simulink model "dynamics_bicycle_model"  (R2017b)
settings: Solver=FixedStepAuto  StartTime=0.0  StopTime=5  FixedStep=0.002  RelTol=1e-3
values from neighbouring files (symbols this model uses):
  af = 1.07    [main_dynamic_bicycle.m]
  ar = 0.936    [main_dynamic_bicycle.m]
  Bf = 0.242    [main_dynamic_bicycle.m]
  Br = 0.24    [main_dynamic_bicycle.m]
  Cf = 1.352    [main_dynamic_bicycle.m]
  Cr = 1.29    [main_dynamic_bicycle.m]
  Df = 2751.69    [main_dynamic_bicycle.m]
  Dr = 3113.08    [main_dynamic_bicycle.m]
  Ef = -0.392    [main_dynamic_bicycle.m]
  Er = 0.507    [main_dynamic_bicycle.m]
  input_type = 3    [main_bicycle.m]    (also in main_differential_steer.m; main_dynamic_bicycle.m)
  Iz = 552.718    [main_dynamic_bicycle.m]
  m = 645    [main_dynamic_bicycle.m]
  r = 0.3    [main_dynamic_bicycle.m]
  theta0 = 0    [main_differential_steer.m]    (also in main_dynamic_bicycle.m)
  v_const = 1    [main_bicycle.m]    (also in main_dynamic_bicycle.m = 0.9)
  v_dot = 0    [main_dynamic_bicycle.m]
  x0 = 0    [main_differential_steer.m]    (also in main_dynamic_bicycle.m)
  y0 = 0    [main_differential_steer.m]    (also in main_dynamic_bicycle.m)
settings Model: Creator=zhenghe3  LastModifiedBy=zhenghe3

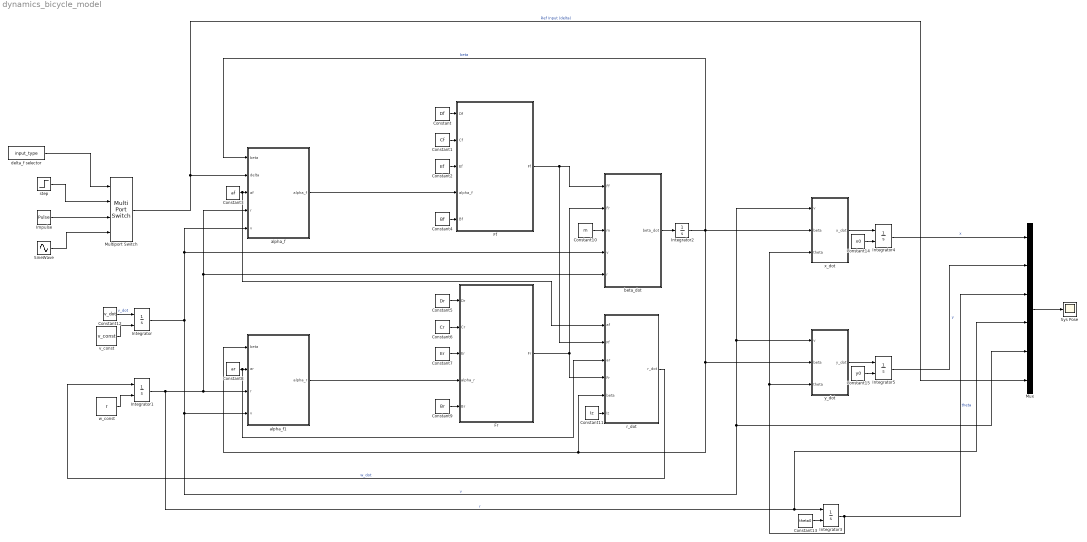
== system dynamics_bicycle_model ==
  Constant : Constant  Value=Df
  Constant1 : Constant  Value=Cf
  Constant10 : Constant  Value=m
  Constant11 : Constant  Value=Iz
  Constant12 : Constant  Value=v_dot
  Constant13 : Constant  Value=theta0
  Constant14 : Constant  Value=x0
  Constant15 : Constant  Value=y0
  Constant2 : Constant  Value=Ef
  Constant3 : Constant  Value=af
  Constant4 : Constant  Value=Bf
  Constant5 : Constant  Value=Dr
  Constant6 : Constant  Value=Cr
  Constant7 : Constant  Value=Er
  Constant8 : Constant  Value=ar
  Constant9 : Constant  Value=Br
  Ff : MATLAB Function  TreatAsAtomicUnit=on
  Fr : MATLAB Function  TreatAsAtomicUnit=on
  Impulse : DiscretePulseGenerator  PulseType=Time based  Period=1  PulseWidth=50
  Integrator{,1,3..5} (5 alike) : Integrator  InitialConditionSource=external
  Integrator2 : Integrator
  Multiport Switch : MultiPortSwitch
  Mux : Mux  Inputs=6
  SineWave : Sin  Frequency=5  SampleTime=0
  Sys Pose : Scope
  alpha_f : MATLAB Function  TreatAsAtomicUnit=on
  alpha_f1 : MATLAB Function  TreatAsAtomicUnit=on
  beta_dot : MATLAB Function  TreatAsAtomicUnit=on
  delta_f selector : Constant  Value=input_type
  r_dot : MATLAB Function  TreatAsAtomicUnit=on
  step : Step  Time=0  SampleTime=0
  v_const : Constant  Value=v_const
  w_const : Constant  Value=r
  x_dot : MATLAB Function  TreatAsAtomicUnit=on
  y_dot : MATLAB Function  TreatAsAtomicUnit=on
  wires:
  Constant12/1 -> Integrator/1  "v_dot"
  Integrator4/1 -> Mux/1  "x"
  Integrator5/1 -> Mux/2  "y"
  Mux/1 -> Sys Pose/1
  v_const/1 -> Integrator/2
  Multiport Switch/1 -> alpha_f/2(delta), Mux/6  "Ref Input (delta)"
  delta_f selector/1 -> Multiport Switch/1
  step/1 -> Multiport Switch/2
  Impulse/1 -> Multiport Switch/3
  SineWave/1 -> Multiport Switch/4
  w_const/1 -> Integrator1/2
  r_dot/1(r_dot) -> Integrator1/1  "w_dot"
  Constant/1 -> Ff/1(Df)
  Constant1/1 -> Ff/2(Cf)
  Constant2/1 -> Ff/3(Ef)
  Constant4/1 -> Ff/5(Bf)
  Constant5/1 -> Fr/1(Dr)
  Constant6/1 -> Fr/2(Cr)
  Constant7/1 -> Fr/3(Er)
  alpha_f1/1(alpha_r) -> Fr/4(alpha_r)
  Constant9/1 -> Fr/5(Br)
  Integrator/1 -> Mux/5, y_dot/1(v), x_dot/1(v), alpha_f1/4(v), beta_dot/4(v), alpha_f/5(v)  "v"
  Integrator1/1 -> Mux/4, Integrator3/1, alpha_f1/3(r), beta_dot/5(r), alpha_f/4(r)  "r"
  Constant3/1 -> r_dot/1(af), alpha_f/3(af)
  Constant8/1 -> r_dot/3(ar), alpha_f1/2(ar)
  alpha_f/1(alpha_f) -> Ff/4(alpha_f)
  Ff/1(Ff) -> r_dot/2(Ff), beta_dot/1(Ff)
  Fr/1(Fr) -> r_dot/4(Fr), beta_dot/2(Fr)
  Constant10/1 -> beta_dot/3(m)
  beta_dot/1(beta_dot) -> Integrator2/1
  Integrator2/1 -> x_dot/2(beta), y_dot/2(beta), r_dot/5(beta), alpha_f1/1(beta), alpha_f/1(beta)  "beta"
  Constant11/1 -> r_dot/6(Iz)
  Constant13/1 -> Integrator3/2
  Integrator3/1 -> y_dot/3(theta), x_dot/3(theta), Mux/3  "theta"
  x_dot/1(x_dot) -> Integrator4/1
  y_dot/1(y_dot) -> Integrator5/1
  Constant14/1 -> Integrator4/2
  Constant15/1 -> Integrator5/2

== matlab function dynamics_bicycle_model/Ff ==
  data: Df input; Ff output; Cf input; Ef input; alpha_f input; Bf input
function Ff = calc_Ff(Df, Cf, Ef, alpha_f, Bf)

Ff = Df * (sin(Cf * atan(Ef * atan(alpha_f * Bf) + (alpha_f * Bf) * (1 - Ef))));

== matlab function dynamics_bicycle_model/Fr ==
  data: Dr input; Fr output; Cr input; Er input; alpha_r input; Br input
function Fr = calc_Fr(Dr, Cr, Er, alpha_r, Br)

Fr = Dr * (sin(Cr * atan(Er * atan(alpha_r * Br) + (alpha_r * Br) * (1 - Er))));

== matlab function dynamics_bicycle_model/alpha_f ==
  data: beta input; alpha_f output; delta input; af input; r input; v input
function alpha_f = calc_alpha_f(beta, delta, af, r, v)

alpha_f = (beta - delta) + atan(af * r * cos(beta) / v);

== matlab function dynamics_bicycle_model/alpha_f1 ==
  data: beta input; alpha_r output; ar input; r input; v input
function alpha_r = calc_alpha_r(beta, ar, r, v)

alpha_r = beta - atan(ar * r * cos(beta) / v);

== matlab function dynamics_bicycle_model/beta_dot ==
  data: Ff input; beta_dot output; Fr input; m input; v input; r input
function beta_dot = calc_beta_dot(Ff, Fr, m, v, r)

beta_dot = (Ff + Fr) / (m * v) - r;

== matlab function dynamics_bicycle_model/r_dot ==
  data: af input; r_dot output; Ff input; ar input; Fr input; beta input; Iz input
function r_dot = calc_r_dot(af, Ff, ar, Fr, beta, Iz)

r_dot = (af*Ff - ar*Fr) * cos(beta) / Iz;

== matlab function dynamics_bicycle_model/x_dot ==
  data: v input; x_dot output; beta input; theta input
function x_dot = calc_x_dot(v, beta, theta)

x_dot = v * cos(beta + theta);

== matlab function dynamics_bicycle_model/y_dot ==
  data: v input; y_dot output; beta input; theta input
function y_dot = calc_y_dot(v, beta, theta)

y_dot = v * sin(beta + theta);
